simulink model "nonlinear_plot"  (Simulink 8.3)
settings: Solver=ode3  StartTime=0.0  StopTime=tf  FixedStep=ts  RelTol=1e-3
values from neighbouring files (symbols this model uses):
  A = 5*(rand(2,1)-0.5)    [phase_plot_Initit.m]
libraries: simulink x1
settings Model: Creator=AMIN  LastModifiedBy=AMIN
settings DataIOCC: SignalLoggingSaveFormat=Dataset
settings DebuggingCC: UnderspecifiedInitializationDetection=Simplified  StateNameClashWarn=none
settings GRTTargetCC: CombineOutputUpdateFcns=on  GRTInterface=off

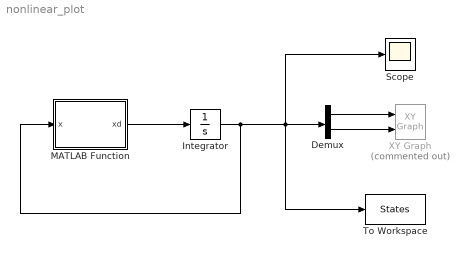
== system nonlinear_plot ==
  Demux : Demux  Outputs=2
  Integrator : Integrator  InitialCondition=A
  MATLAB Function : MATLAB Function  TreatAsAtomicUnit=on
  Scope : Scope
  To Workspace : ToWorkspace  VariableName=States  SampleTime=-1
  XY Graph : simulink/Sinks/XY Graph  Commented=on  xmin=-1  xmax=1  ymin=-1  ymax=1  st=-1
  wires:
  MATLAB Function/1(xd) -> Integrator/1
  Integrator/1 -> MATLAB Function/1(x), Scope/1, Demux/1, To Workspace/1
  Demux/1 -> XY Graph/1
  Demux/2 -> XY Graph/2

== matlab function MATLAB Function ==
  data: x input double; xd output double
function xd = Dyn(x)
x1 = x(1);
x2 = x(2);
%% Define Sys States here + dynamics
%% A %%
%  x1d = x2;
%  x2d = -x2-0.5*x1;

%% B %%
% x1d = x2;
% x2d = 1-x2-0.5*x1;

%% C %%
% x1d = x2;
% x2d = -x2.^2-0.5*x1;
%% Problem 4 %%
b = 0.5;
x1d = -x1+0.1*x2+(x1^2)*x2;
x2d = b-0.1*x2-(x1^2)*x2;

%% %%
xd = [x1d;x2d];
end
